simulink model "pcm2"  (R2017a)
settings: Solver=VariableStepAuto  StartTime=0.0  StopTime=50  MaxStep=1e-4  RelTol=1e-3
libraries: commchan3 x1, dsparch4 x1, dspsigops x1
settings Model: Creator=Vibha  LastModifiedBy=Vibha

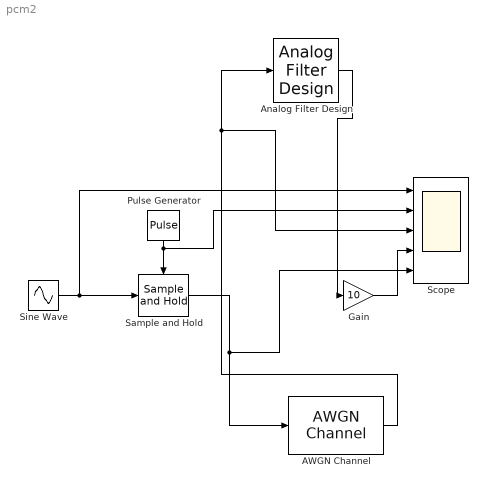
== system pcm2 ==
  AWGN Channel : commchan3/AWGN Channel  InputProcessing=Columns as channels (frame based)  seed=67  noiseMode=Variance from mask  EbNodB=10  EsNodB=10  SNRdB=10  bitsPerSym=1  Ps=1  Tsym=1  variance=30
  Analog Filter Design : dsparch4/Analog Filter Design  method=Butterworth  filttype=Lowpass  N=8  Wlo=3.5*pi  Whi=3.5*pi  Rp=2  Rs=40
  Gain : Gain  Gain=10
  Pulse Generator : DiscretePulseGenerator  PulseType=Time based  Period=0.1  PulseWidth=5
  Sample and Hold : dspsigops/Sample and Hold  trig=Rising edge  initCond=0  latchinput=off
  Scope : Scope  NumInputPorts=5
  Sine Wave : Sin  Frequency=2*pi  SampleTime=0
  wires:
  Analog Filter Design/1 -> Gain/1
  Gain/1 -> Scope/4
  Sine Wave/1 -> Scope/1, Sample and Hold/1
  Pulse Generator/1 -> Scope/2, Sample and Hold/Trigger
  Sample and Hold/1 -> Scope/5, AWGN Channel/1
  AWGN Channel/1 -> Scope/3, Analog Filter Design/1
